simulink model "tune"  (R2022a)
settings: Solver=FixedStepAuto  StartTime=0.0  StopTime=inf  RelTol=1e-3
libraries: vexv5lib x2, slctrlblks x1, slpidlib x1
settings Model: Creator=chpfoxtrot  LastModifiedBy=chpfoxtrot
settings OptimizationCC: EnhancedBackFolding=on  PassReuseOutputArgsAs=Individual arguments  ZeroExternalMemoryAtStartup=off  ZeroInternalMemoryAtStartup=off  MaxStackSize=64  OptimizeBlockOrder=speed  DifferentSizesBufferReuse=on  OptimizationCustomize=off  EfficientTunableParamExpr=on
settings DebuggingCC: ParameterTunabilityLossMsg=error
settings HardwareCC: ProdBitPerPointer=32  ProdBitPerSizeT=32  ProdBitPerPtrDiffT=32  ProdLargestAtomicInteger=Long  ProdLargestAtomicFloat=Double  ProdWordSize=32  ProdHWDeviceType=ARM Compatible->ARM Cortex  UseEmbeddedCoderFeatures=off
settings SFSimCC: MATLABDynamicMemAlloc=off
settings RTWCC: SystemTargetFile=ert.tlc  HardwareBoard=VEX V5 Robot Brain  TLCOptions="-aInlineSetEventsForThisBaseRateFcn=TLC_FALSE -aSuppressMultiTaskScheduler=TLC_FALSE  -aRateBasedStepFcn=0"  TemplateMakefile=ert_default_tmf  Toolchain=GNU Tools for ARM Embedded Processors
settings CodeAppCC: ForceParamTrailComments=on  IgnoreCustomStorageClasses=off  OperatorAnnotations=on  SimulinkDataObjDesc=on  SFDataObjDesc=on  InsertBlockDesc=on
settings ERTTargetCC: SupportNonInlinedSFcns=on  ExtModeTransport=3  ExtModeStaticAlloc=on  ExtModeStaticAllocSize=2048  ExtModeMexFile=ext_xcp  ExtModeIntrfLevel=Level2 - Open

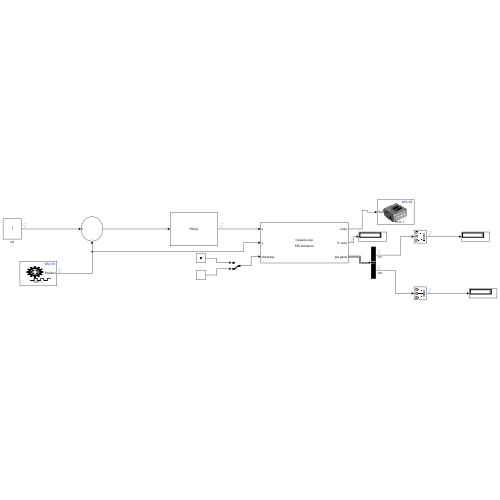
[thumbnail: Simulink's stored preview of the top-level diagram]
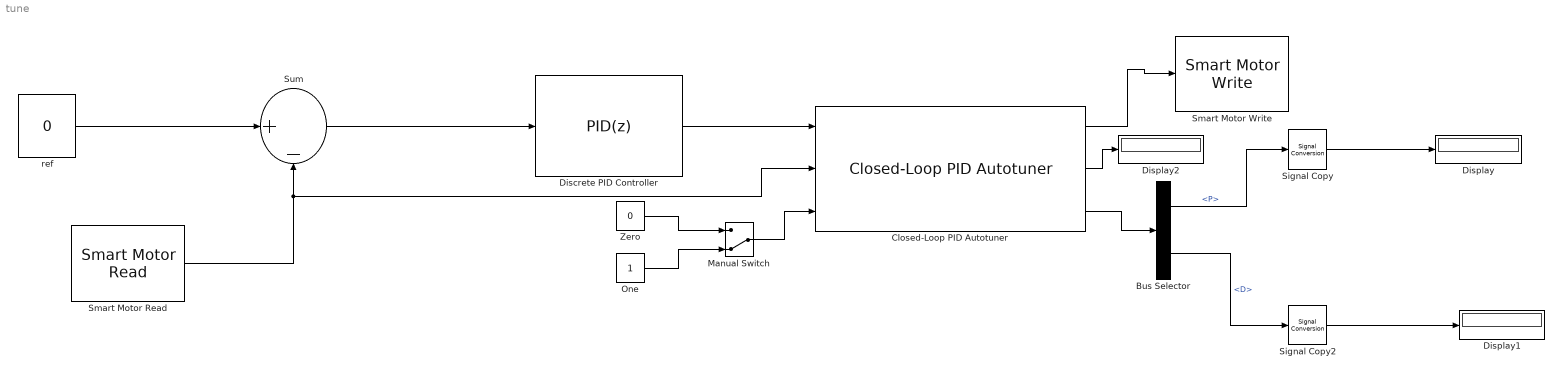
== system tune ==
  Bus Selector : BusSelector  OutputSignals=P,D
  Closed-Loop PID Autotuner : slctrlblks/Closed-Loop PID Autotuner  PIDType=PD  PIDForm=Parallel  TimeDomain=discrete-time  DiscreteTs=0.02  TuningTs=0.2  UseTuningTs=off  IntegratorFormula=Forward Euler  FilterFormula=Forward Euler  ContinuousTs=0.02  Bandwidth=2*6.28  UseExternalWC=off  TargetPM=60  UseExternalPM=off  UseExternalAchievedPM=off  ExperimentMode=Superposition  PlantType=Stable  PlantSign=Positive  AmpSine=10  UseExternalAmpSine=off  UseExternalFRD=off  UseExternalU0=off  UseCompanion=off  NotDeployTuningModule=off  UsePLCCoder=off  OutputMode=control action + perturbation  BlockDataType=double  UseConnectedPID=on  blockpath=[]  tunedP=0  tunedI=0  tunedD=0  tunedN=100  tunedPM=0  EstimationWindowSize=3  UseExternalTuningParams=off  OutputChoice=VariantCandD  SingleMultiRateVariant=SingleSamplingRate  ExperimentModeVariant=VariantSuperimposed  NumEstimationPeriods=4  NumSettlingPeriods=2
      settings: SourceProductBaseCode=SD
  Discrete PID Controller : slpidlib/PID Controller  Controller=PID  Form=Parallel  TimeDomain=Discrete-time  UseExternalTs=off  SampleTime=-1  IntegratorMethod=Forward Euler  FilterMethod=Forward Euler  ControllerParametersSource=internal  P=1  I=1  UseKiTs=off  D=0  N=100  UseFilter=on  TunerSelectOption=Transfer Function Based (PID Tuner App)  InitialConditionSource=internal  InitialConditionForIntegrator=0  InitialConditionForFilter=0  DifferentiatorICPrevScaledInput=0  ExternalReset=none  TrackingMode=off  Kt=1  LimitOutput=off  SatLimitsSource=internal  UpperSaturationLimit=inf  LowerSaturationLimit=-inf  LinearizeAsGain=off  AntiWindupMode=none  Kb=1  POutMin=[]  POutMax=[]  IOutMin=[]  IOutMax=[]  DOutMin=[]  DOutMax=[]  NOutMin=[]  NOutMax=[]  SumOutMin=[]  SumOutMax=[]  SaturationOutMin=[]  SaturationOutMax=[]  PParamMin=[]  PParamMax=[]  IParamMin=[]  IParamMax=[]  DParamMin=[]  DParamMax=[]  NParamMin=[]  NParamMax=[]  KbParamMin=[]  KbParamMax=[]  KtParamMin=[]  KtParamMax=[]  KbOutMin=[]  KbOutMax=[]  KtOutMin=[]  KtOutMax=[]  IntegratorOutMin=[]  IntegratorOutMax=[]  FilterOutMin=[]  FilterOutMax=[]  SumI1OutMin=[]  SumI1OutMax=[]  SumI2OutMin=[]  SumI2OutMax=[]  SumI3OutMin=[]  SumI3OutMax=[]  SumI4OutMin=[]  SumI4OutMax=[]  SumDOutMin=[]  SumDOutMax=[]  DifferentiatorOutMin=[]  DifferentiatorOutMax=[]  FilterDiffOutCoefMin=[]  FilterDiffOutCoefMax=[]  ReciprocalOutMin=[]  ReciprocalOutMax=[]  SumDenOutMin=[]  SumDenOutMax=[]  SumNumOutMin=[]  SumNumOutMax=[]  DivideOutMin=[]  DivideOutMax=[]  UdiffTsProdOutMin=[]  UdiffTsProdOutMax=[]  NTsProdOutMin=[]  NTsProdOutMax=[]  UintegralTsProdOutMin=[]  UintegralTsProdOutMax=[]  UngainTsProdOutMin=[]  UngainTsProdOutMax=[]  IntegratorContinuousStateAttributes=''  IntegratorStateMustResolveToSignalObject=off  IntegratorRTWStateStorageClass=Auto  FilterContinuousStateAttributes=''  FilterStateMustResolveToSignalObject=off  FilterRTWStateStorageClass=Auto  ParallelPVariant=InternalParameters  IdealPVariant=Disabled  IVariant=InternalParameters  DVariant=InternalParameters  IntegratorVariant=Discrete  SatVariant=Disabled  AWVariant=Passthrough  PCopyVariant=Disabled  TRVariant=Disabled  FdbkBlocksVariant=Forward  IdealPFdbkVariant=Disabled  SatFdbkVariant=Disabled  DerivativeFilterVariant=ForwardEulerFilter  NVariant=InternalParameters  NCopyVariant=Disabled  FilterICVariant=InternalICsFilter  IntegratorICVariant=InternalICs  ExternalResetVariant=Disabled  TRSumVariant=Passthrough  SumFdbkVariant=Disabled  SumVariant=Sum_PID  TsampFilterVariant=InternalTs  TsampNgainVariant=Passthrough  TsampIntegralVariant=Passthrough  ExternalSaturationOutDataTypeStr=Inherit: Same as second input  aMode=0
  Display : Display
  Display1 : Display
  Display2 : Display
  Manual Switch : ManualSwitch  CurrentSetting=0
  One : Constant  OutDataTypeStr=Inherit: Inherit via back propagation
  Signal Copy : SignalConversion  OverrideOpt=off
  Signal Copy2 : SignalConversion  OverrideOpt=off
  Smart Motor Read : vexv5lib/Sensors/Smart Motor Read  motorPort=1  EncoderUnit=Counts  resetOption=No reset  additionalOutput=off  SampleTime=0.2
      settings: SourceProductBaseCode=VEXV5
  Smart Motor Write : vexv5lib/Actuators/Smart Motor Write  motorPort=1  scaleFactor=18:1  MotorBrakeMode=Coast  OperationMode=Velocity Control
      settings: SourceProductBaseCode=VEXV5
  Sum : Sum  Inputs=|+-
  Zero : Constant  Value=0  OutDataTypeStr=Inherit: Inherit via back propagation
  ref : Constant  Value=0
  wires:
  ref/1 -> Sum/1
  Discrete PID Controller/1 -> Closed-Loop PID Autotuner/1
  Manual Switch/1 -> Closed-Loop PID Autotuner/3
  Zero/1 -> Manual Switch/1
  One/1 -> Manual Switch/2
  Closed-Loop PID Autotuner/3 -> Bus Selector/1
  Bus Selector/2 -> Signal Copy2/1  "<D>"
  Bus Selector/1 -> Signal Copy/1  "<P>"
  Signal Copy2/1 -> Display1/1
  Signal Copy/1 -> Display/1
  Smart Motor Read/1 -> Closed-Loop PID Autotuner/2, Sum/2
  Closed-Loop PID Autotuner/1 -> Smart Motor Write/1
  Closed-Loop PID Autotuner/2 -> Display2/1
  Sum/1 -> Discrete PID Controller/1
